simulink model "demo6_1"  (R2018b)
settings: Solver=FixedStepAuto  StartTime=0.0  StopTime=1800  FixedStep=0.01  RelTol=1e-3
libraries: simulink x2
settings Model: Creator=Gavin  LastModifiedBy=Gavin
settings OptimizationCC: DefaultParameterBehavior=Inlined  EnhancedBackFolding=on  PassReuseOutputArgsAs=Individual arguments  OptimizeBlockOrder=speed  DifferentSizesBufferReuse=on  OptimizationCustomize=off
settings DebuggingCC: ParameterTunabilityLossMsg=error
settings SFSimCC: MATLABDynamicMemAlloc=off
settings RTWCC: SystemTargetFile=ert.tlc  TemplateMakefile=ert_default_tmf  GenerateReport=on  IncludeHyperlinkInReport=on  LaunchReport=on  GenerateTraceInfo=on  GenerateTraceReport=on  GenerateTraceReportSl=on  GenerateTraceReportSf=on  GenerateTraceReportEml=on
settings CodeAppCC: ForceParamTrailComments=on  IgnoreCustomStorageClasses=off  OperatorAnnotations=on  SimulinkDataObjDesc=on  SFDataObjDesc=on  InsertBlockDesc=on
settings ERTTargetCC: TargetLangStandard=C99 (ISO)  GenerateSampleERTMain=on  InlinedParameterPlacement=NonHierarchical  ERTCustomFileTemplate=example_file_process.tlc

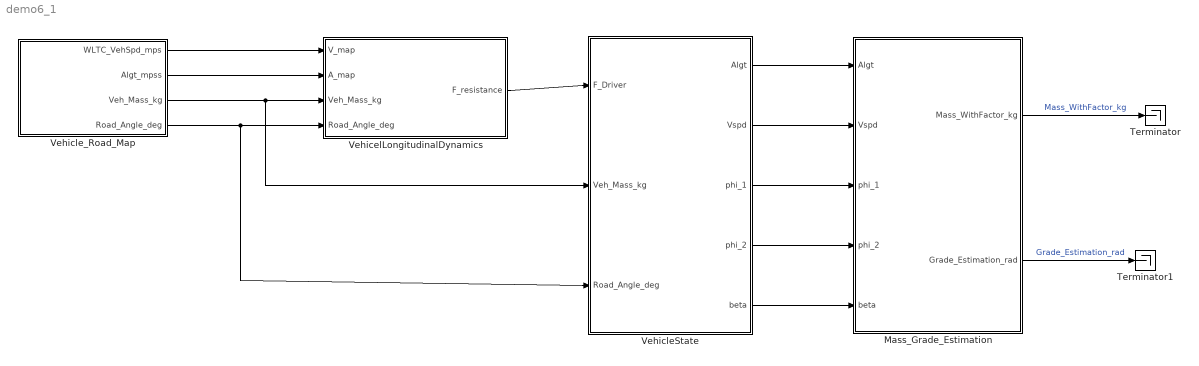
== system demo6_1 ==
  Mass_Grade_Estimation : Subsystem
  Terminator : Terminator
  Terminator1 : Terminator
  VehicelLongitudinalDynamics : Subsystem
  VehicleState : Subsystem
  Vehicle_Road_Map : Subsystem
  wires:
  Vehicle_Road_Map/1(WLTC_VehSpd_mps) -> VehicelLongitudinalDynamics/1(V_map)
  Vehicle_Road_Map/2(Algt_mpss) -> VehicelLongitudinalDynamics/2(A_map)
  Vehicle_Road_Map/3(Veh_Mass_kg) -> VehicleState/2(Veh_Mass_kg), VehicelLongitudinalDynamics/3(Veh_Mass_kg)
  Vehicle_Road_Map/4(Road_Angle_deg) -> VehicleState/3(Road_Angle_deg), VehicelLongitudinalDynamics/4(Road_Angle_deg)
  VehicelLongitudinalDynamics/1(F_resistance) -> VehicleState/1(F_Driver)
  VehicleState/1(Algt) -> Mass_Grade_Estimation/1(Algt)
  VehicleState/2(Vspd) -> Mass_Grade_Estimation/2(Vspd)
  VehicleState/3(phi_1) -> Mass_Grade_Estimation/3(phi_1)
  VehicleState/4(phi_2) -> Mass_Grade_Estimation/4(phi_2)
  VehicleState/5(beta) -> Mass_Grade_Estimation/5(beta)
  Mass_Grade_Estimation/1(Mass_WithFactor_kg) -> Terminator/1  "Mass_WithFactor_kg"
  Mass_Grade_Estimation/2(Grade_Estimation_rad) -> Terminator1/1  "Grade_Estimation_rad"

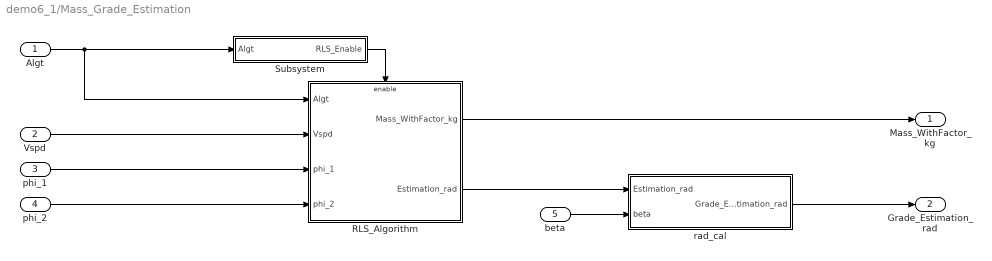
== system demo6_1/Mass_Grade_Estimation ==
  Algt : Inport
  Vspd : Inport  Port=2
  phi_1 : Inport  Port=3
  phi_2 : Inport  Port=4
  beta : Inport  Port=5
  RLS_Algorithm : Subsystem
  Subsystem : Subsystem
  rad_cal : Subsystem
  Mass_WithFactor_kg : Outport
  Grade_Estimation_rad : Outport  Port=2
  wires:
  phi_2/1 -> RLS_Algorithm/4(phi_2)
  phi_1/1 -> RLS_Algorithm/3(phi_1)
  Vspd/1 -> RLS_Algorithm/2(Vspd)
  RLS_Algorithm/1(Mass_WithFactor_kg) -> Mass_WithFactor_kg/1
  Algt/1 -> RLS_Algorithm/1(Algt), Subsystem/1(Algt)
  Subsystem/1(RLS_Enable) -> RLS_Algorithm/Enable
  RLS_Algorithm/2(Estimation_rad) -> rad_cal/1(Estimation_rad)
  beta/1 -> rad_cal/2(beta)
  rad_cal/1(Grade_Estimation_rad) -> Grade_Estimation_rad/1

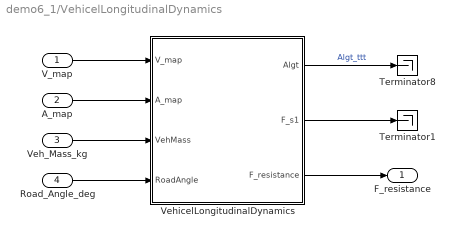
== system demo6_1/VehicelLongitudinalDynamics ==
  V_map : Inport
  A_map : Inport  Port=2
  Veh_Mass_kg : Inport  Port=3
  Road_Angle_deg : Inport  Port=4
  Terminator1 : Terminator
  Terminator8 : Terminator
  VehicelLongitudinalDynamics : MATLAB Function  TreatAsAtomicUnit=on
  F_resistance : Outport
  wires:
  VehicelLongitudinalDynamics/1(Algt) -> Terminator8/1  "Algt_ttt"
  Road_Angle_deg/1 -> VehicelLongitudinalDynamics/4(RoadAngle)
  VehicelLongitudinalDynamics/3(F_resistance) -> F_resistance/1
  A_map/1 -> VehicelLongitudinalDynamics/2(A_map)
  V_map/1 -> VehicelLongitudinalDynamics/1(V_map)
  VehicelLongitudinalDynamics/2(F_s1) -> Terminator1/1
  Veh_Mass_kg/1 -> VehicelLongitudinalDynamics/3(VehMass)

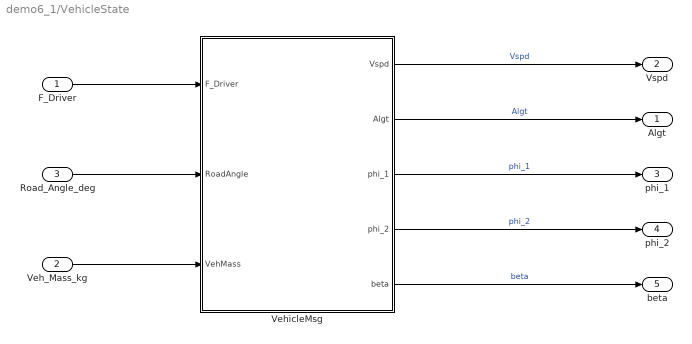
== system demo6_1/VehicleState ==
  F_Driver : Inport
  Veh_Mass_kg : Inport  Port=2
  Road_Angle_deg : Inport  Port=3
  VehicleMsg : MATLAB Function  TreatAsAtomicUnit=on
  Algt : Outport
  Vspd : Outport  Port=2
  phi_1 : Outport  Port=3
  phi_2 : Outport  Port=4
  beta : Outport  Port=5
  wires:
  Veh_Mass_kg/1 -> VehicleMsg/3(VehMass)
  VehicleMsg/2(Algt) -> Algt/1  "Algt"
  VehicleMsg/1(Vspd) -> Vspd/1  "Vspd"
  VehicleMsg/5(beta) -> beta/1  "beta"
  Road_Angle_deg/1 -> VehicleMsg/2(RoadAngle)
  VehicleMsg/3(phi_1) -> phi_1/1  "phi_1"
  F_Driver/1 -> VehicleMsg/1(F_Driver)
  VehicleMsg/4(phi_2) -> phi_2/1  "phi_2"

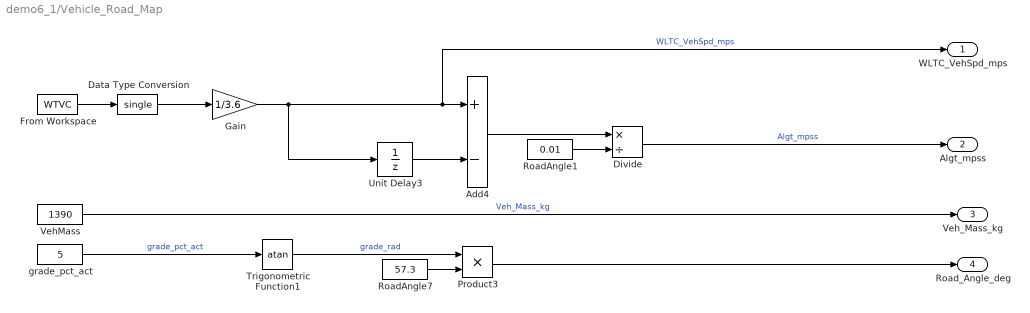
== system demo6_1/Vehicle_Road_Map ==
  Add4 : Sum  Inputs=+-
  Data Type Conversion : DataTypeConversion  OutDataTypeStr=single
  Divide : Product  Inputs=*/
  From Workspace : FromWorkspace  VariableName=WTVC  SampleTime=0
  Gain : Gain  Gain=1/3.6
  Product3 : Product
  RoadAngle1 : Constant  Value=0.01  OutDataTypeStr=single
  RoadAngle7 : Constant  Value=57.3  OutDataTypeStr=single
  Trigonometric Function1 : Trigonometry  Operator=atan
  Unit Delay3 : UnitDelay  SampleTime=-1
  VehMass : Constant  Value=1390  OutDataTypeStr=single
  grade_pct_act : Constant  Value=5  OutDataTypeStr=single
  WLTC_VehSpd_mps : Outport
  Algt_mpss : Outport  Port=2
  Veh_Mass_kg : Outport  Port=3
  Road_Angle_deg : Outport  Port=4
  wires:
  Gain/1 -> Unit Delay3/1, WLTC_VehSpd_mps/1, Add4/1  "WLTC_VehSpd_mps"
  RoadAngle1/1 -> Divide/2
  Unit Delay3/1 -> Add4/2
  From Workspace/1 -> Data Type Conversion/1
  Add4/1 -> Divide/1
  Divide/1 -> Algt_mpss/1  "Algt_mpss"
  Product3/1 -> Road_Angle_deg/1
  Trigonometric Function1/1 -> Product3/1  "grade_rad"
  grade_pct_act/1 -> Trigonometric Function1/1  "grade_pct_act"
  RoadAngle7/1 -> Product3/2
  VehMass/1 -> Veh_Mass_kg/1  "Veh_Mass_kg"
  Data Type Conversion/1 -> Gain/1

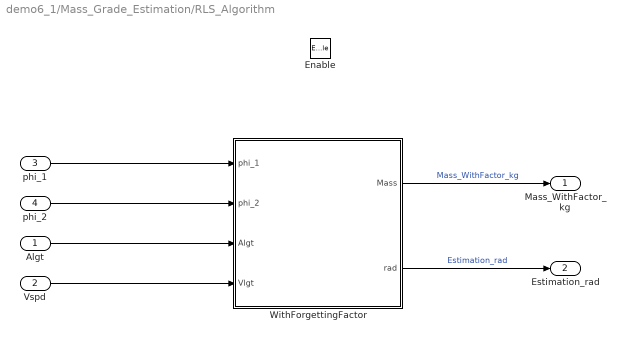
== system demo6_1/Mass_Grade_Estimation/RLS_Algorithm ==
  Algt : Inport
  Vspd : Inport  Port=2
  phi_1 : Inport  Port=3
  phi_2 : Inport  Port=4
  Enable : EnablePort
  WithForgettingFactor : MATLAB Function  TreatAsAtomicUnit=on
  Mass_WithFactor_kg : Outport  InitialOutput=1500
  Estimation_rad : Outport  Port=2
  wires:
  Algt/1 -> WithForgettingFactor/3(Algt)
  phi_1/1 -> WithForgettingFactor/1(phi_1)
  phi_2/1 -> WithForgettingFactor/2(phi_2)
  Vspd/1 -> WithForgettingFactor/4(Vlgt)
  WithForgettingFactor/2(rad) -> Estimation_rad/1  "Estimation_rad"
  WithForgettingFactor/1(Mass) -> Mass_WithFactor_kg/1  "Mass_WithFactor_kg"

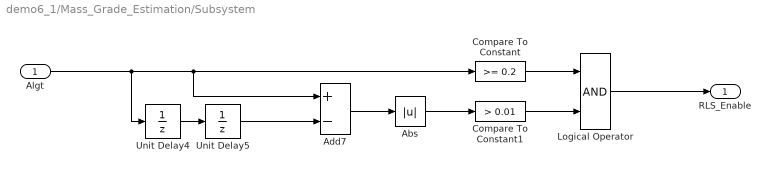
== system demo6_1/Mass_Grade_Estimation/Subsystem ==
  Algt : Inport
  Abs : Abs
  Add7 : Sum  Inputs=+-
  Compare To Constant : simulink/Logic and Bit Operations/Compare To Constant  relop=>=  const=0.2  OutDataTypeStr=boolean
  Compare To Constant1 : simulink/Logic and Bit Operations/Compare To Constant  relop=>  const=0.01  OutDataTypeStr=boolean
  Logical Operator : Logic  AllPortsSameDT=off  OutDataTypeStr=boolean
  Unit Delay4 : UnitDelay  SampleTime=-1
  Unit Delay5 : UnitDelay  SampleTime=-1
  RLS_Enable : Outport
  wires:
  Logical Operator/1 -> RLS_Enable/1
  Abs/1 -> Compare To Constant1/1
  Add7/1 -> Abs/1
  Unit Delay5/1 -> Add7/2
  Compare To Constant1/1 -> Logical Operator/2
  Unit Delay4/1 -> Unit Delay5/1
  Algt/1 -> Compare To Constant/1, Add7/1, Unit Delay4/1
  Compare To Constant/1 -> Logical Operator/1

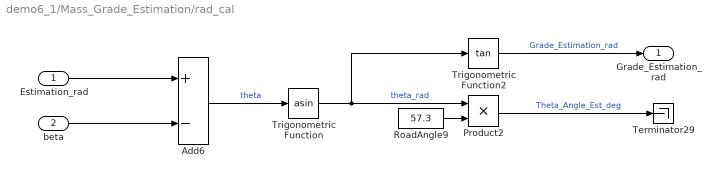
== system demo6_1/Mass_Grade_Estimation/rad_cal ==
  Estimation_rad : Inport
  beta : Inport  Port=2
  Add6 : Sum  Inputs=+-
  Product2 : Product
  RoadAngle9 : Constant  Value=57.3
  Terminator29 : Terminator
  Trigonometric Function : Trigonometry  Operator=asin
  Trigonometric Function2 : Trigonometry  Operator=tan
  Grade_Estimation_rad : Outport
  wires:
  beta/1 -> Add6/2
  Trigonometric Function/1 -> Trigonometric Function2/1, Product2/1  "theta_rad"
  Trigonometric Function2/1 -> Grade_Estimation_rad/1  "Grade_Estimation_rad"
  Product2/1 -> Terminator29/1  "Theta_Angle_Est_deg"
  RoadAngle9/1 -> Product2/2
  Add6/1 -> Trigonometric Function/1  "theta"
  Estimation_rad/1 -> Add6/1

== matlab function demo6_1/VehicelLongitudinalDynamics/VehicelLongitudinalDynamics ==
  data: V_map input; A_map input; VehMass input; RoadAngle input; Algt output; F_s1 output; F_resistance output
function [Algt ,F_s1,F_resistance]   = VehLgtDyn(V_map,A_map,VehMass,RoadAngle)
% This function is vehicle longitudinal dynamics
% By Du QingYa
persistent a_buff
if isempty(a_buff)
    a_buff = A_map;
end
V = V_map;
g = single(9.8);
r = single(0.3638); % tryers radius
A_Cd = single(0.3); %aerodynamic drag coefficient
front_ares = single(2.38); 
air_density = single(1.1567);
% VehMass = 1390;
% RoadAngle = 0/180;
Ration = single(9.7);


% Vehicle gradient resistance force define
f_grad =single(VehMass * g * sin(RoadAngle*pi/180));
% Rolling resistance force define
Crr = single(0.01 * (1 + (V./100)));
f_r = single(Crr * VehMass * g * cos(RoadAngle*pi/180));
% Aerodynamic resistance force define
f_a = single(0.5 * air_density * front_ares * A_Cd * V.^2);
% Inertia resistance force define
f_i = single(1.15 * VehMass * A_map);

% Cal Actual Speed(m/s) and Acceleration

F_resistance = VehMass*A_map +  f_grad + f_r + f_a;

% a1 = g * sin(RoadAngle/180) + A_map;
f_r1 = Crr * VehMass * g;
F_s1 = f_r1 + f_a + VehMass*A_map;

P_driver = single(F_resistance .* V/1000);
v1 = single(V * 3.6);
Algt = F_resistance / VehMass;
a_buff = Algt;

== matlab function demo6_1/VehicleState/VehicleMsg ==
  settings: updateMethod=DISCRETE
  data: F_Driver input; Vspd output; RoadAngle input; VehMass input; Algt output; phi_1 output; phi_2 output; beta output
function [Vspd,Algt,phi_1,phi_2,beta] = VehLgtDyn(F_Driver,RoadAngle,VehMass)

persistent v_buff
if isempty(v_buff)
v_buff = single(0);
end
g = single(9.8);
% r = 0.3638; % tryers radius
A_Cd = single(0.3); %aerodynamic drag coefficient
front_ares = single(2.38); 
air_density = single(1.1567);
% VehMass = 1390;
% RoadAngle = 0/180;
% Ration = 9.7;


% Vehicle gradient resistance force define
f_grad = single(VehMass * g * sin(RoadAngle*pi/180));
% Rolling resistance force define
Crr = single(0.01 * (1 + (v_buff/100)));
f_r = single(Crr * VehMass * g * cos(RoadAngle*pi/180));
% Aerodynamic resistance force define
f_a = single(0.5 * air_density * front_ares * A_Cd * v_buff^2);
% Inertia resistance force define
% f_i = 1.15 * VehMass * a_buff;

F_forward = F_Driver - f_a - f_grad - f_r;
phi_1 = F_Driver - f_a;
beta = atan(Crr );
phi_2 = -g/cos(beta);
% syb = sign(F_forward);
a_buff = F_forward / VehMass;
v_buff = single(v_buff + a_buff * 0.01);


Algt = a_buff; %No g vector
Vspd = v_buff;


end

== matlab function demo6_1/Mass_Grade_Estimation/RLS_Algorithm/WithForgettingFactor ==
  settings: updateMethod=DISCRETE
  data: phi_1 input; phi_2 input; Mass output; Algt input; Vlgt input; rad output
function [Mass, rad]= MassEstimation(phi_1,phi_2,Algt,Vlgt)
% RLS of Estimation Vehicle Mass and Slope
% By Du QingYa
persistent x P
if isempty(x)
    x = cast([1/1400;0],class(Vlgt));  % state variables initial
    P = cast([0.0001 0;0 0.01],class(Vlgt)); % covariance matrix
end
%     H = g * sin(0) + 0.01 * (1 + Vlgt ./ 100) * g*cos(0) + 1.15 * Algt;
%     H = 1.15 * Algt + g * 0.01 * (1 + Vlgt ./ 100);
    H =[phi_1,phi_2];
    Z =Algt;
    Lamda =single(0.95);
    K = P*H'/(H*P*H' + Lamda);
    P = (eye(2) - K*H)*P/Lamda;           % covariance matrix P update
    x = x+K*(Z-H*x);               % x state update
    
    Mass = 1/x(1,1);
    rad = x(2);
%     road_rad = rad - beta;
%     angle = 180 * road_rad/pi;
end
